simulink model "READ_UAL_POSE"  (R2018a)
settings: Solver=VariableStepAuto  StartTime=0.0  StopTime=10.0  RelTol=1e-3
libraries: robotlib x1
settings Model: Creator=root  LastModifiedBy=root

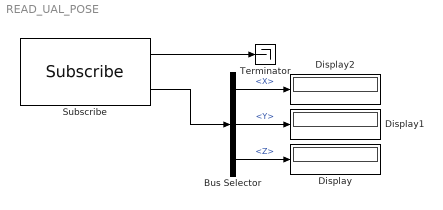
== system READ_UAL_POSE ==
  Bus Selector : BusSelector  OutputSignals=Pose.Position.X,Pose.Position.Y,Pose.Position.Z
  Display : Display
  Display1 : Display
  Display2 : Display
  Subscribe : robotlib/Subscribe  SourceLibraryInfo=This block requires Robotics System Toolbox  topicSource=Select from ROS network  topic=/ual/pose  messageType=geometry_msgs/PoseStamped  sampleTime=inf  messageQueueLength=1
      settings: SourceProductBaseCode=RO
  Terminator : Terminator
  wires:
  Subscribe/2 -> Bus Selector/1
  Bus Selector/3 -> Display/1  "<Z>"
  Bus Selector/1 -> Display2/1  "<X>"
  Bus Selector/2 -> Display1/1  "<Y>"
  Subscribe/1 -> Terminator/1
